simulink model "ekf6_grp3"  (R2018b)
settings: Solver=ode5  StartTime=0.0  StopTime=1800  FixedStep=0.1  MaxStep=0.1  RelTol=1e-3  AbsTol=1e-6
StartFcn:
  | clear radarLogsOut
StopFcn:
  | aero_radplot;
model workspace (MATLAB code in the model file):
  | g = 32.2;    % Acceleration due to gravity (ft/sec^2)
  | tauc = 5;    % Correlation time of aircraft cross axis acceleration
  | tauT = 4;    % Correlation time of aircraft thrust axis acceleration
  | Speed = 400; % Initial speed of aircraft in y direction feet/sec
  | deltat = 1;  % Radar update rate (also hard-coded in extkalman.m)
libraries: simulink x2
CloseFcn:
  | h=findobj('type','figure');if ~isempty(h);close(h);end
  | clear radarLogsOut
  | clear h;
Description:
  | Radar Tracking Using MATLAB Function Block
  | 
  | This example shows how to use an extended Kalman filter with the
  | MATLAB(R) Function block in Simulink(R) to estimate an aircraft's
  | position from radar measurements. The filter implementation is found in the
  | MATLAB Function block, the contents of which are stored in the
  | Simulink model itself.
  | 
  | At the end of the simulation, three figures display the following information: the
  | actual trajectory compared to the estimated trajectory; the estimation residual
  | for range; and the actual, measured, and estimated positions.
settings Model: ExtModeTrigMode=oneshot  ExtModeArmWhenConnect=off  ExtModeAutoUpdateStatusClock=off  Creator=The MathWorks, Inc.  LastModifiedBy=1star
settings SolverCC: AutoScaleAbsTol=off
settings DataIOCC: SaveFormat=Array  SaveOutput=off  SaveTime=off  TimeSaveName=t_sim  SignalLoggingName=radarLogsOut
settings OptimizationCC: DefaultParameterBehavior=Inlined  InlineInvariantSignals=on  ExpressionDepthLimit=2147483647  StateBitsets=on  DataBitsets=on  ZeroExternalMemoryAtStartup=off  ZeroInternalMemoryAtStartup=off  NoFixptDivByZeroProtection=on  LifeSpan=1  BufferReusableBoundary=off
settings DebuggingCC: SaveWithParameterizedLinksMsg=none  CheckExecutionContextPreStartOutputMsg=on  CheckExecutionContextRuntimeOutputMsg=on  SignalResolutionControl=TryResolveAllWithWarning  MultiTaskDSMMsg=warning  MultiTaskCondExecSysMsg=none  FcnCallInpInsideContextMsg=warning  StateNameClashWarn=warning  SFUnexpectedBacktrackingDiag=warning  SFNoUnconditionalDefaultTransitionDiag=warning  SFExecutionAtInitializationDiag=none
settings HardwareCC: ProdBitPerPointer=32  ProdBitPerSizeT=32  ProdBitPerPtrDiffT=32  ProdLargestAtomicFloat=None  ProdIntDivRoundTo=Undefined  ProdEndianess=Unspecified  ProdWordSize=32  ProdHWDeviceType=32-bit Generic
settings ModelReferenceCC: PropagateSignalLabelsOutOfModel=off
settings SFSimCC: SimUseLocalCustomCode=off  SimParseCustomCode=off  MATLABDynamicMemAlloc=off
settings RTWCC: SystemTargetFile=ert.tlc  TLCOptions=-p0 -aWarnNonSaturatedBlocks=0  TemplateMakefile=ert_default_tmf  Description=RTW Embedded Coder (no auto configuration)  GenerateReport=on  RTWVerbose=off  RTWUseLocalCustomCode=off  IncludeHyperlinkInReport=on  LaunchReport=on
settings CodeAppCC: ForceParamTrailComments=on  IgnoreCustomStorageClasses=off  SimulinkDataObjDesc=on  CustomSymbolStrType=$N$R$M  CustomSymbolStrFcn=$F$N$M  CustomSymbolStrMacro=$N$M  InsertBlockDesc=on  StateflowObjectComments=on  InternalIdentifier=Classic
settings ERTTargetCC: TargetFcnLib=ansi_tfl_tmw.mat  MultiwordLength=2048  GenerateSampleERTMain=on  IncludeMdlTerminateFcn=off  SupportComplex=off  SupportContinuousTime=on  SupportNonInlinedSFcns=on  InlinedParameterPlacement=NonHierarchical  ERTCustomFileTemplate=example_file_process.tlc  ConvertIfToSwitch=off  SuppressUnreachableDefaultCases=off
settings ConfigComp: CovMetricSettings=d  CovHtmlReporting=on  CovSaveCumulativeToWorkspaceVar=on  CovSaveSingleToWorkspaceVar=on  CovExternalEMLEnable=off

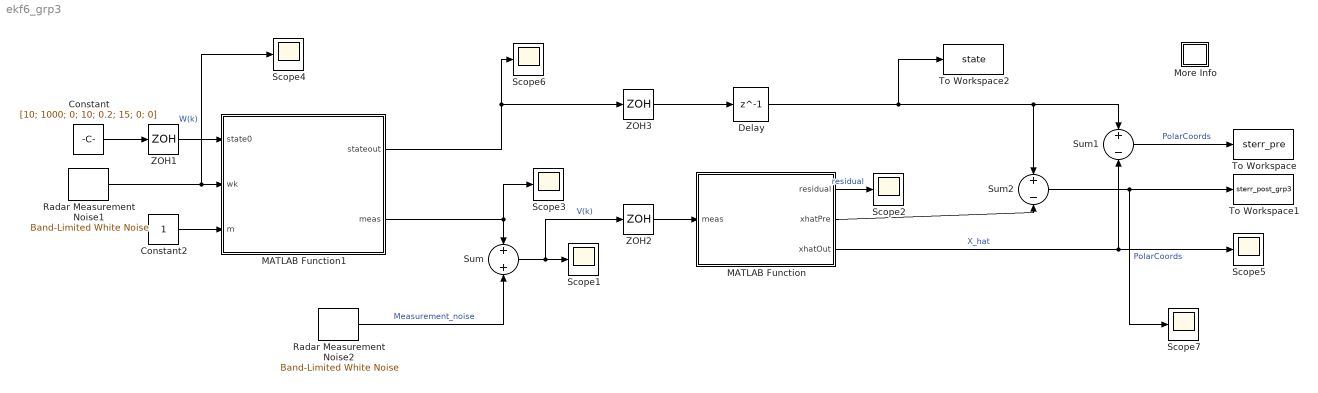
== system ekf6_grp3 ==
  Constant : Constant  Value=[10; 1000; 0; 10; 0.2; 15; 0; 0]  SampleTime=deltat
  Constant2 : Constant  SampleTime=0.1
  Delay : Delay  DelayLength=1  InitialCondition=0
  MATLAB Function : MATLAB Function  TreatAsAtomicUnit=on
  MATLAB Function1 : MATLAB Function  TreatAsAtomicUnit=on
  More Info : Subsystem
      settings: OpenFcn=showdemo(bdroot(gcs))
      mask Display: disp('?')
  Radar Measurement Noise1 : simulink/Sources/Band-Limited White Noise  Cov=[0 0 0 0 0 0 0 0]  Ts=0.1  seed=[52341; 62341; 72341; 82341; 92341; 10341; 11341; 12341]
  Radar Measurement Noise2 : simulink/Sources/Band-Limited White Noise  Cov=[1 4]  Ts=0.1  seed=[52341 62341]
  Scope{1..7} (7 alike) : Scope
  Sum : Sum  Inputs=2  SaturateOnIntegerOverflow=on  InputSameDT=on  OutDataTypeStr=Inherit: Same as first input
  Sum1 : Sum  Inputs=+-  SaturateOnIntegerOverflow=on  InputSameDT=on  OutDataTypeStr=Inherit: Same as first input
  Sum2 : Sum  Inputs=+-  SaturateOnIntegerOverflow=on  InputSameDT=on  OutDataTypeStr=Inherit: Same as first input
  To Workspace : ToWorkspace  VariableName=sterr_pre  SampleTime=-1
  To Workspace1 : ToWorkspace  VariableName=sterr_post_grp3  SampleTime=-1
  To Workspace2 : ToWorkspace  VariableName=state  SampleTime=-1
  ZOH1 : ZeroOrderHold  SampleTime=0.1
  ZOH2 : ZeroOrderHold  SampleTime=0.5
  ZOH3 : ZeroOrderHold  SampleTime=0.5
  wires:
  MATLAB Function/1(residual) -> Scope2/1  "residual"
  MATLAB Function/3(xhatOut) -> Sum1/2, Scope5/1  "X_hat"
  MATLAB Function1/2(meas) -> Sum/1, Scope3/1
  Radar Measurement Noise2/1 -> Sum/2  "Measurement_noise"
  MATLAB Function1/1(stateout) -> Scope6/1, ZOH3/1
  Sum/1 -> ZOH2/1, Scope1/1  "V(k)"
  Constant/1 -> ZOH1/1
  ZOH1/1 -> MATLAB Function1/1(state0)
  Radar Measurement Noise1/1 -> Scope4/1, MATLAB Function1/2(wk)  "W(k)"
  Constant2/1 -> MATLAB Function1/3(m)
  ZOH2/1 -> MATLAB Function/1(meas)
  ZOH3/1 -> Delay/1
  MATLAB Function/2(xhatPre) -> Sum2/2
  Sum2/1 -> To Workspace1/1, Scope7/1  "PolarCoords"
  Sum1/1 -> To Workspace/1  "PolarCoords"
  Delay/1 -> To Workspace2/1, Sum2/1, Sum1/1

== system ekf6_grp3/More Info ==

== matlab function ekf6_grp3/MATLAB Function1 ==
  data: state0 input double; wk input; m input; stateout output double; meas output
function [stateout, meas]  = Envrionment(state0, wk, m)
%EXTKALMAN Radar Data Processing Tracker Using an Extended Kalman Filter
%
%  This program is executed as a MATLAB function block in the 
%  sldemo_radar Simulink model.  The estimated and actual positions are 
%  saved to the workspace and are plotted at the end of the simulation by 
%  the program aero_radplot (called from the simulation automatically).
%
%

%  Copyright 1990-2013 The MathWorks, Inc.

% Initialization
deltat = 0.1;
g=9.836;
maxstep=50;

persistent step;
persistent index;
persistent state;
if isempty(index)
    index = 0;
end
if isempty(state)
    state = state0;
end
if isempty(step)
    step=0;
end
if index==0 
    state = state0;
%     state(5)=state0(5)*(9+2*step/maxstep)/10;
%     state(6)=state0(6)*(9+2*step/maxstep)/10;
%     state(7)=state0(5)*(9+2*step/maxstep)/10;
%     state(8)=state0(6)*(9+2*step/maxstep)/10;
    state(5)=state0(5)*step/maxstep;
    state(6)=state0(6)*step/maxstep;
    state(7)=state0(5)*step/maxstep;
    state(8)=state0(6)*step/maxstep;
end

 
h_ = 2;
bet_ = 150;
rho0_ = 1.225;
kp_ = 9200;
% 
ry = state(2);
vy = state(4);
deltah = state(5);
deltabet = state(6);
deltarho = state(7);
deltakp = state(8);
% 
h=h_+deltah;
bet=bet_+deltabet;
rho0=rho0_+deltarho;
kp=kp_+deltakp;
% 
alpha = rho0*exp(-ry/kp)*vy*vy/(2*m*bet);
% 
phi = [1 0 deltat 0 0 0 0 0; 0 1 0 deltat 0 0 0 0; 0 0 1 0 0 0 0 0; 0 -alpha*deltat/kp 0 1+rho0*exp(-ry/kp)*vy/(m*bet)*deltat 0 -alpha/bet*deltat alpha/rho0*deltat ry*alpha*deltat/(kp*kp);
    0 0 0 0 1 0 0 0; 0 0 0 0 0 1 0 0; 0 0 0 0 0 0 1 0; 0 0 0 0 0 0 0 1];
u = [0; -g*deltat*deltat/2; 0; -g*deltat*(1+rho0*exp(-ry/kp)*vy/(2*m*bet)); 0; 0; 0; 0];

state = phi*state + u + wk;

% 
H = [1 0 0 0 0 0 0 0; 0 1 0 0 0 0 0 0];
b = [0; -h];
y = H*state + b;

meas = y;
index = index+1;
if(index==360)
    index=0;
    step=step+1;
end

stateout = state;

== matlab function ekf6_grp3/MATLAB Function ==
  data: meas input double; residual output double; xhatPre output; xhatOut output double
function [residual, xhatPre ,xhatOut] = EXTKALMAN(meas)
%EXTKALMAN Radar Data Processing Tracker Using an Extended Kalman Filter
%
%  This program is executed as a MATLAB function block in the 
%  sldemo_radar Simulink model.  The estimated and actual positions are 
%  saved to the workspace and are plotted at the end of the simulation by 
%  the program aero_radplot (called from the simulation automatically).
%
%

%  Copyright 1990-2013 The MathWorks, Inc.

% Initialization
maxstep = 50;

persistent step;
persistent index;
persistent P;
persistent xhat;

if isempty(index)
    index = 0;
end

if isempty(P)
    xhat = [0; 1000; 0; 0; 0; 0; 0; 0];
    P = zeros(8);
    P(2)=10;
    P(4)=1;   
end

if isempty(step)
    step=0;
end

if(index==0) 
    xhat = [0; 1000; 0; 0; 0; 0; 0; 0];
    P = diag([0 0 10 10 0 0 0 0])*(9.5+step/maxstep)/10;
end

g=9.836;
delta_t=0.5;
m = 1;
h_ = 2;
bet_ = 150;
rho0_ = 1.225;
kp_ = 9200;
% 
ry = xhat(2);
vy = xhat(4);
deltah = xhat(5);
deltabet = xhat(6);
deltarho = xhat(7);
deltakp = xhat(8);
% 
h=h_+deltah;
bet=bet_+deltabet;
rho0=rho0_+deltarho;
kp=kp_+deltakp;
% 
alpha = rho0*exp(-ry/kp)*vy*vy/(2*m*bet);
% 
% 1. Compute Phi, Q, and R 
Phi = [1 0 delta_t 0 0 0 0 0; 0 1 0 delta_t 0 0 0 0; 0 0 1 0 0 0 0 0; 0 -alpha*delta_t/kp 0 1+rho0*exp(-ry/kp)*vy/(m*bet)*delta_t 0 -alpha/bet*delta_t alpha/rho0*delta_t ry*alpha*delta_t/(kp*kp);
    0 0 0 0 1 0 0 0; 0 0 0 0 0 1 0 0; 0 0 0 0 0 0 1 0; 0 0 0 0 0 0 0 1];
Q =  diag([1 10 0.01 1 0 0 0 0]);
R =  diag([1 4]);

% 2. Propagate the covariance matrix:
P = Phi*P*Phi' + Q;

% 3. Propagate the track estimate::
u = [0; -g*delta_t*delta_t/2; 0; -g*delta_t*(1+rho0*exp(-ry/kp)*vy/(2*m*bet)); 0; 0; 0; 0];
xhat = Phi*xhat+u;
xhatPre = xhat;
% 4 a). Compute observation estimates:
H = [1 0 0 0 0 0 0 0; 0 1 0 0 0 0 0 0];
b = [0; -h];
yhat = H*xhat + b;

% 4 c).  Compute residual (Estimation Error)
residual = meas - yhat;

% 5. Compute Kalman Gain:
W = P*H'*inv(H*P*H'+ R);
% 
% % 6. Update estimate
xhat = xhat + W*residual;
% 
% % 7. Update Covariance Matrix
P = (eye(8)-W*H)*P*(eye(8)-W*H)' + W*R*W';

index=index+1;
if(index==72)
    index=0;
    step=step+1;
end

xhatOut = xhat;
